simulink model "lecture05_12"  (R2020a)
settings: Solver=VariableStepAuto  StartTime=0.0  StopTime=10.0  RelTol=1e-3
values from neighbouring files (symbols this model uses):
  Acl = A-B*K    [lecture05_11.m]    (also in lecture05_8.m)
  Aov = A-L*C    [lecture05_10.m]    (also in lecture05_11.m)
  Bcl = B*K*Nx    [lecture05_11.m]    (also in lecture05_8.m)
  Bov = [B L]    [lecture05_10.m]    (also in lecture05_11.m)
  Ccl = C    [lecture05_11.m]    (also in lecture05_8.m)
  Cov = eye(2)    [lecture05_10.m]    (also in lecture05_11.m)
  Dcl = D*K*Nx    [lecture05_11.m]    (also in lecture05_8.m)
  Dov = Cov*Bov*0    [lecture05_10.m]    (also in lecture05_11.m)
  K = tf(numK, denK)    [lecture02_5.m]    (also in lecture05_1.m = Kp+Kd+Ki/s; lecture05_11.m = place(A,B,p); lecture05_2.m = Kp+Kd+Ki/s; lecture05_3.m = Kp+Kd+Ki/s)
settings Model: Creator=JY  LastModifiedBy=JY

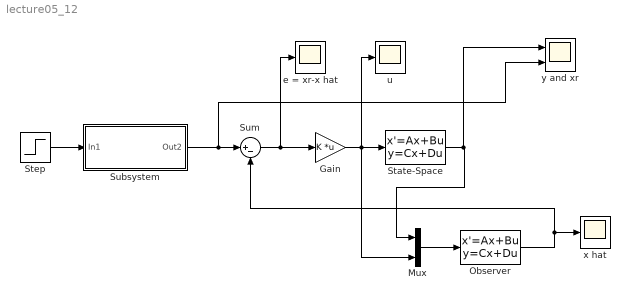
== system lecture05_12 ==
  Gain : Gain  Gain=K  Multiplication=Matrix(K*u)
  Mux : Mux  Inputs=2
  Observer : StateSpace  A=Aov  B=Bov  C=Cov  D=Dov  InitialCondition=0
  State-Space : StateSpace  A=Acl  B=Bcl  C=Ccl  D=Dcl  InitialCondition=0
  Step : Step  SampleTime=0
  Subsystem : Subsystem
  Sum : Sum  Inputs=|+-
  e = xr-x hat : Scope
  u : Scope
  x hat : Scope
  y and xr : Scope  NumInputPorts=2
  wires:
  Step/1 -> Subsystem/1(In1)
  Gain/1 -> Mux/2, u/1, State-Space/1
  State-Space/1 -> y and xr/1, Mux/1
  Subsystem/1(Out2) -> y and xr/2, Sum/1
  Sum/1 -> e = xr-x hat/1, Gain/1
  Mux/1 -> Observer/1
  Observer/1 -> Sum/2, x hat/1

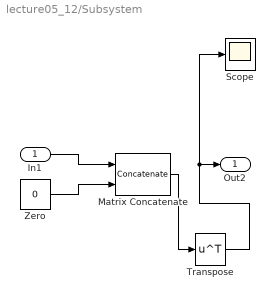
== system lecture05_12/Subsystem ==
  In1 : Inport
  Matrix Concatenate : Concatenate  Mode=Multidimensional array  ConcatenateDimension=2
  Scope : Scope
  Transpose : Math  Operator=transpose  SaturateOnIntegerOverflow=on
  Zero : Constant  Value=0  OutDataTypeStr=Inherit: Inherit via back propagation
  Out2 : Outport
  wires:
  In1/1 -> Matrix Concatenate/1
  Zero/1 -> Matrix Concatenate/2
  Matrix Concatenate/1 -> Transpose/1
  Transpose/1 -> Scope/1, Out2/1
